simulink model "sim1"  (R2024a)
settings: Solver=FixedStepAuto  StartTime=0.0  StopTime=22.0  FixedStep=1  RelTol=1e-3
settings Model: Creator=alexe  LastModifiedBy=alexe

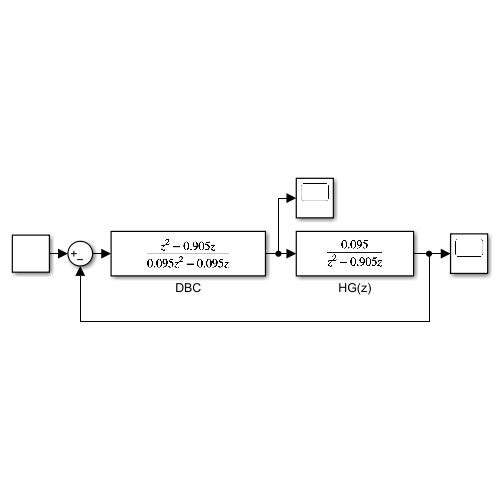
[thumbnail: Simulink's stored preview of the top-level diagram]
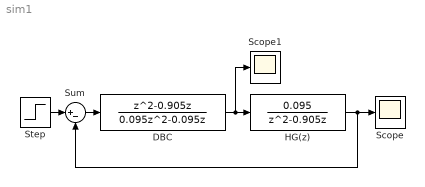
== system sim1 ==
  DBC : DiscreteTransferFcn  Numerator=[1 -0.905 0]  Denominator=[0.095 -0.095 0]
  HG(z) : DiscreteTransferFcn  Numerator=[0 0 0.095]  Denominator=[1 -0.905 0]
  Scope : Scope
  Scope1 : Scope
  Step : Step  Time=3  SampleTime=0
  Sum : Sum  Inputs=|+-
  wires:
  Step/1 -> Sum/1
  Sum/1 -> DBC/1
  DBC/1 -> Scope1/1, HG(z)/1
  HG(z)/1 -> Sum/2, Scope/1
